simulink subsystem "Parameters"  (R2022a)
settings: Solver=VariableStepAuto  StartTime=0.0  StopTime=10.0  RelTol=1e-3
undefined symbols (not defined in the file): ACT_THRESH, ACTIVITY_THRESH, AMP, ATR_DURATION, ATR_FALLBACK_MODE, ATR_FALLBACK_TIME, BATTERY_VOLTAGE, D0, D1, D13, D3, D6, DYNAMIC_AV_DELAY, FIXED_AV_DELAY, HYSTERESIS, LEAD_IMPEDANCE, LRL, MAX_SENSOR_RATE, P_WAVE, PTA1, PTC16, PTC17, PTC2, PTD1, PULSE_WIDTH, PVARP, PVARP_EXT, R_WAVE, RATE_SMOOTHING, REACTION_TIME, RECOVERY_TIME, RESPONSE_FACTOR, RP, SENSED_AV_DELAY_OFFSET, SENSITIVITY, URL
libraries: frdmk64flib x8, simulink x1
settings Model: Creator=bkfre  LastModifiedBy=bkfre

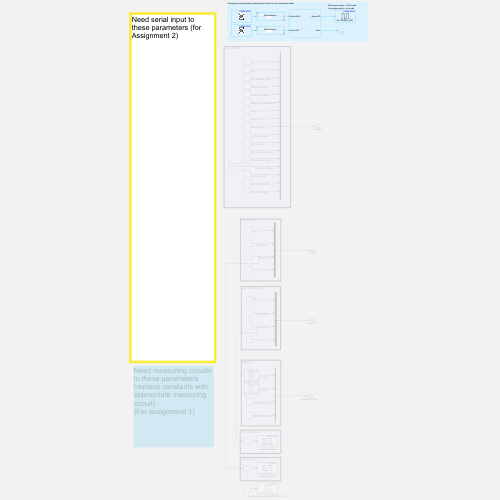
[thumbnail: Simulink's stored preview of the top-level diagram]
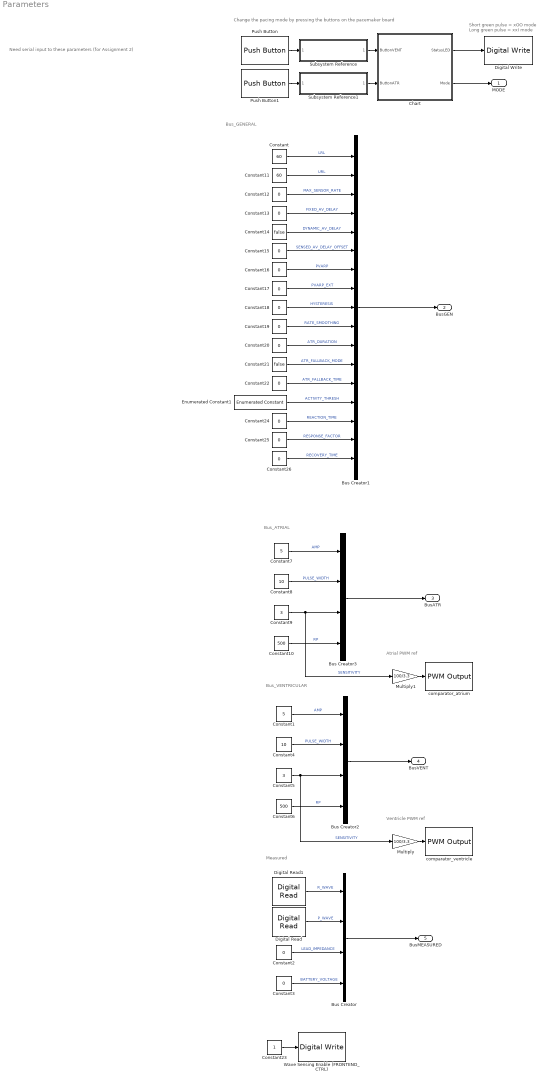
== system Parameters ==
  note: Short green pulse = xOO mode
      | Long green pulse = xxI mode
  note: Change the pacing mode by pressing the buttons on the pacemaker board
  note: Need serial input to these parameters (for Assignment 2)
  note: Bus_ATRIAL
  note: Bus_VENTRICULAR
  note: Measured
  note: Bus_GENERAL
  note: Ventricle PWM ref
  note: Atrial PWM ref
  Bus Creator : BusCreator  Inputs=R_WAVE,P_WAVE,LEAD_IMPEDANCE,BATTERY_VOLTAGE  OutDataTypeStr=Bus: BusMEASURED  NonVirtualBus=on
  Bus Creator1 : BusCreator  Inputs=LRL,URL,MAX_SENSOR_RATE,FIXED_AV_DELAY,DYNAMIC_AV_DELAY,SENSED_AV_DELAY_OFFSET,PVARP,PVARP_EXT,HYSTERESIS,RATE_SMOOTHING,ATR_DURATION,ATR_FALLBACK_MODE,ATR_FALLBACK_TIME,ACTIVITY_THRESH,REACTION_TIME,RESPONSE_FACTOR,RECOVERY_TIME  OutDataTypeStr=Bus: BusGEN  NonVirtualBus=on
  Bus Creator2 : BusCreator  Inputs=AMP,PULSE_WIDTH,SENSITIVITY,RP  OutDataTypeStr=Bus: BusSPECIFIC  NonVirtualBus=on
  Bus Creator3 : BusCreator  Inputs=AMP,PULSE_WIDTH,SENSITIVITY,RP  OutDataTypeStr=Bus: BusSPECIFIC  NonVirtualBus=on
  Chart : Stateflow chart  TreatAsAtomicUnit=on
  Constant : Constant  Value=60
  Constant1 : Constant  Value=5
  Constant10 : Constant  Value=500
  Constant11 : Constant  Value=60
  Constant{2..3,12..13,15..19,22,24..26} (13 alike) : Constant  Value=0
  Constant14 : Constant  Value=false  OutDataTypeStr=boolean
  Constant20 : Constant  Value=0  OutDataTypeStr=int64
  Constant21 : Constant  Value=false  OutDataTypeStr=boolean
  Constant23 : Constant  SampleTime=-1
  Constant4 : Constant  Value=10
  Constant5 : Constant  Value=3
  Constant6 : Constant  Value=500
  Constant7 : Constant  Value=5
  Constant8 : Constant  Value=10
  Constant9 : Constant  Value=3
  Digital Read : frdmk64flib/Digital Read  Whichpin=PTC16 (D0)  SampleTime=-1
  Digital Read1 : frdmk64flib/Digital Read  Whichpin=PTC17 (D1)  SampleTime=-1
  Digital Write : frdmk64flib/Digital Write  Whichpin=GREEN_LED
  Enumerated Constant1 : simulink/Sources/Enumerated Constant  OutDataTypeStr=Enum: ACT_THRESH  Value=ACT_THRESH.VLOW  SampleTime=inf
  Multiply : Gain  Gain=100/3.3
  Multiply1 : Gain  Gain=100/3.3
  Push Button : frdmk64flib/Push Button  Whichswitch=SW2  SampleTime1=-1
  Push Button1 : frdmk64flib/Push Button  Whichswitch=SW3  SampleTime1=-1
  Subsystem Reference : Subsystem  ReferencedSubsystem=BtnDebounce
  Subsystem Reference1 : Subsystem  ReferencedSubsystem=BtnDebounce
  Wave Sensing Enable (FRONTEND_CTRL) : frdmk64flib/Digital Write  Whichpin=PTD1 (D13)
  comparator_atrium : frdmk64flib/PWM Output  Whichpin=PTC2 (D6)  InitialFrequency=2000  InitialDutyCycle=0
  comparator_ventricle : frdmk64flib/PWM Output  Whichpin=PTA1 (D3)  InitialFrequency=2000  InitialDutyCycle=0
  MODE : Outport  OutDataTypeStr=Enum: MODE
  BusGEN : Outport  Port=2  OutDataTypeStr=Bus: BusGEN
  BusATR : Outport  Port=3  OutDataTypeStr=Bus: BusSPECIFIC
  BusVENT : Outport  Port=4  OutDataTypeStr=Bus: BusSPECIFIC
  BusMEASURED : Outport  Port=5  OutDataTypeStr=Bus: BusMEASURED
  wires:
  Constant7/1 -> Bus Creator3/1  "AMP"
  Constant10/1 -> Bus Creator3/4  "RP"
  Constant8/1 -> Bus Creator3/2  "PULSE_WIDTH"
  Constant9/1 -> Bus Creator3/3, Multiply1/1  "SENSITIVITY"
  Constant6/1 -> Bus Creator2/4  "RP"
  Constant5/1 -> Bus Creator2/3, Multiply/1  "SENSITIVITY"
  Constant1/1 -> Bus Creator2/1  "AMP"
  Constant4/1 -> Bus Creator2/2  "PULSE_WIDTH"
  Constant3/1 -> Bus Creator/4  "BATTERY_VOLTAGE"
  Constant2/1 -> Bus Creator/3  "LEAD_IMPEDANCE"
  Constant26/1 -> Bus Creator1/17  "RECOVERY_TIME"
  Enumerated Constant1/1 -> Bus Creator1/14  "ACTIVITY_THRESH"
  Constant17/1 -> Bus Creator1/8  "PVARP_EXT"
  Constant25/1 -> Bus Creator1/16  "RESPONSE_FACTOR"
  Constant19/1 -> Bus Creator1/10  "RATE_SMOOTHING"
  Constant12/1 -> Bus Creator1/3  "MAX_SENSOR_RATE"
  Constant24/1 -> Bus Creator1/15  "REACTION_TIME"
  Constant22/1 -> Bus Creator1/13  "ATR_FALLBACK_TIME"
  Constant20/1 -> Bus Creator1/11  "ATR_DURATION"
  Constant13/1 -> Bus Creator1/4  "FIXED_AV_DELAY"
  Constant18/1 -> Bus Creator1/9  "HYSTERESIS"
  Constant16/1 -> Bus Creator1/7  "PVARP"
  Constant15/1 -> Bus Creator1/6  "SENSED_AV_DELAY_OFFSET"
  Constant14/1 -> Bus Creator1/5  "DYNAMIC_AV_DELAY"
  Constant21/1 -> Bus Creator1/12  "ATR_FALLBACK_MODE"
  Constant11/1 -> Bus Creator1/2  "URL"
  Constant/1 -> Bus Creator1/1  "LRL"
  Bus Creator3/1 -> BusATR/1
  Bus Creator2/1 -> BusVENT/1
  Bus Creator/1 -> BusMEASURED/1
  Bus Creator1/1 -> BusGEN/1
  Chart/2(Mode) -> MODE/1
  Multiply/1 -> comparator_ventricle/1
  Multiply1/1 -> comparator_atrium/1
  Constant23/1 -> Wave Sensing Enable (FRONTEND_CTRL)/1
  Digital Read1/1 -> Bus Creator/1  "R_WAVE"
  Digital Read/1 -> Bus Creator/2  "P_WAVE"
  Push Button/1 -> Subsystem Reference/1
  Push Button1/1 -> Subsystem Reference1/1
  Chart/1(StatusLED) -> Digital Write/1
  Subsystem Reference/1 -> Chart/1(ButtonVENT)
  Subsystem Reference1/1 -> Chart/2(ButtonATR)

== stateflow chart Parameters/Chart ==
  note: Left Button / SW3 switches between atrial modes
      | Right button / SW2 switches between ventricle modes
  state AOO
    entry:
    Mode=MODE.AOO;
    StatusLED=false;
    state LED_OFF
      entry:
      StatusLED=false;
    state Flash
      entry:
      StatusLED=true;
    (default) -> AOO.Flash
    AOO.Flash -> AOO.LED_OFF : after(100,msec)
  state VOO
    entry:
    Mode=MODE.VOO;
    state LED_OFF
      entry:
      StatusLED=false;
    state Flash
      entry:
      StatusLED=true;
    (default) -> VOO.Flash
    VOO.Flash -> VOO.LED_OFF : after(100,msec)
  state VVI
    entry:
    Mode=MODE.VVI;
    StatusLED=true;
    state LED_OFF
      entry:
      StatusLED=false;
    state Flash
      entry:
      StatusLED=true;
    (default) -> VVI.Flash
    VVI.Flash -> VVI.LED_OFF : after(500,msec)
  state AAI
    entry:
    Mode=MODE.AAI;
    StatusLED=true;
    state LED_OFF
      entry:
      StatusLED=false;
    state Flash
      entry:
      StatusLED=true;
    (default) -> AAI.Flash
    AAI.Flash -> AAI.LED_OFF : after(500,msec)
  (default) -> VOO
  AOO -> VOO [order 2] : [ButtonVENT]
  VOO -> AOO [order 1] : [ButtonATR]
  AOO -> AAI [order 1] : [ButtonATR]
  AAI -> AOO [order 2] : [ButtonATR]
  VOO -> VVI [order 2] : [ButtonVENT]
  VVI -> VOO [order 1] : [ButtonVENT]
  VVI -> AAI [order 2] : [ButtonATR]
  AAI -> VVI [order 1] : [ButtonVENT]
  data: ButtonVENT input; ButtonATR input; StatusLED output boolean; Mode output Enum: MODE
